simulink model "SISO_Sim_c"  (R2015b)
settings: Solver=VariableStepAuto  StartTime=0.0  StopTime=15  RelTol=1e-3
libraries: simulink_extras x2, simulink x1
settings Model: Creator=dmartin_a  LastModifiedBy=dmartin_a

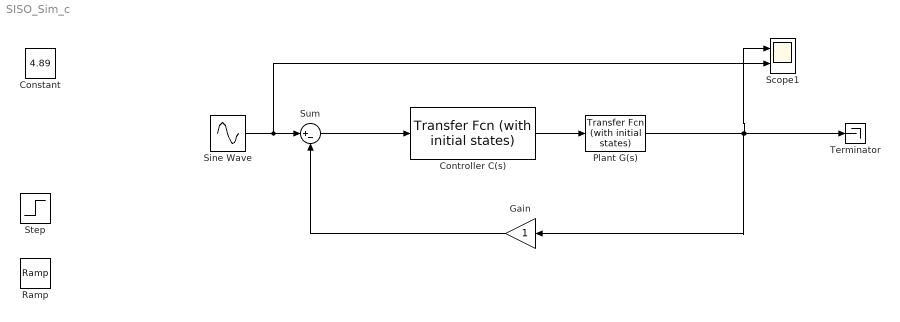
== system SISO_Sim_c ==
  Constant : Constant  Value=4.89  SampleTime=.01
  Controller C(s) : simulink_extras/Additional Linear/Transfer Fcn (with initial states)  N=[1 -6223.39 -25319.5]  D=[1 1892 1]  X0=0
  Gain : Gain
  Plant G(s) : simulink_extras/Additional Linear/Transfer Fcn (with initial states)  N=[-316]  D="[1  -976]"  X0=0
  Ramp : simulink/Sources/Ramp  slope=2  start=5  X0=0
  Scope1 : Scope  NumInputPorts=2
  Sine Wave : Sin  Amplitude=200  SampleTime=0
  Step : Step  SampleTime=0
  Sum : Sum  Inputs=|+-
  Terminator : Terminator
  wires:
  Controller C(s)/1 -> Plant G(s)/1
  Sum/1 -> Controller C(s)/1
  Plant G(s)/1 -> Terminator/1, Scope1/1, Gain/1
  Sine Wave/1 -> Scope1/2, Sum/1
  Gain/1 -> Sum/2
